simulink model "CHB_3phase_Phaseshift"  (R2015a)
settings: Solver=ode45  StartTime=0.0  StopTime=0.06  MaxStep=0.000001  MinStep=0.0000001  RelTol=1e-3
libraries: powerlib x33, powerlib_meascontrol x1, simulink x1
settings Model: Creator=hp  LastModifiedBy=hp

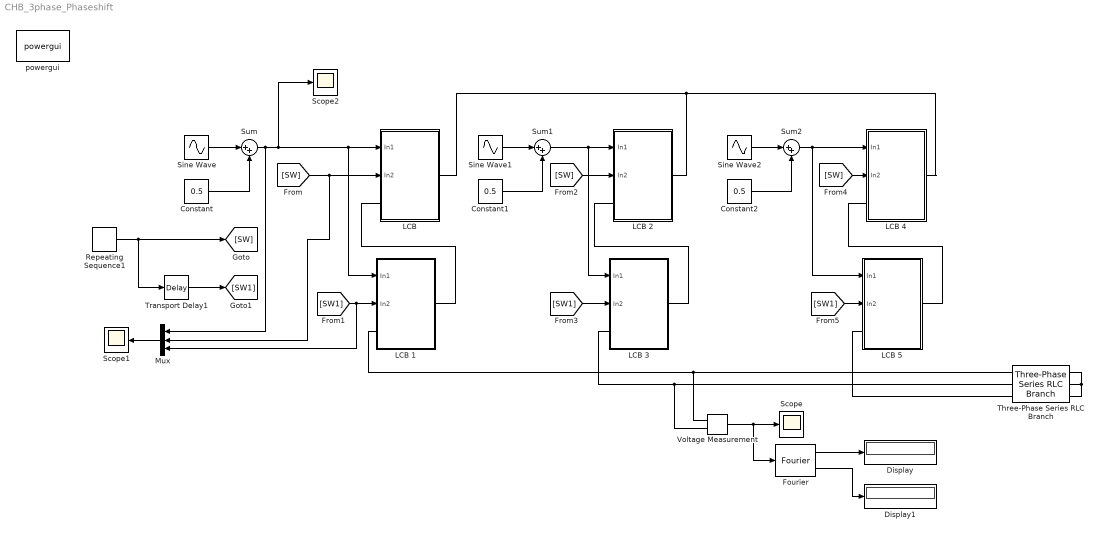
== system CHB_3phase_Phaseshift ==
  Constant : Constant  Value=0.5
  Constant1 : Constant  Value=0.5
  Constant2 : Constant  Value=0.5
  Display : Display
  Display1 : Display
  Fourier : powerlib_meascontrol/Measurements/Fourier  Freq=50  n=1  InInit=[0, 0]  Ts=0
  "LCB " : Subsystem
  LCB 1 : Subsystem
  LCB 2 : Subsystem
  LCB 3 : Subsystem
  LCB 4 : Subsystem
  LCB 5 : Subsystem
  Mux : Mux  Inputs=3
  Repeating Sequence1 : simulink/Sources/Repeating Sequence  rep_seq_t=[0 0.5 1]/1000  rep_seq_y=[0 1 0]
  Scope : Scope
      settings: YMin=-400  YMax=400
  Scope1 : Scope
      settings: YMin=2.77556e-17  YMax=1  SaveName=ScopeData2
  Scope2 : Scope
      settings: YMin=2.77556e-17  YMax=1  SaveName=ScopeData3
  Sine Wave : Sin  Amplitude=0.5  Frequency=2*pi*50  SampleTime=0
  Sine Wave1 : Sin  Amplitude=0.5  Frequency=2*pi*50  Phase=2*pi/3  SampleTime=0
  Sine Wave2 : Sin  Amplitude=0.5  Frequency=2*pi*50  Phase=4*pi/3  SampleTime=0
  Sum : Sum  Inputs=|++
  Sum1 : Sum  Inputs=|++
  Sum2 : Sum  Inputs=|++
  Three-Phase Series RLC Branch : powerlib/Elements/Three-Phase Series RLC Branch  LConnTagsString=A|B|C  RConnTagsString=A|B|C  BranchType=RLC  Resistance=1000  Inductance=0  Capacitance=0  Measurements=None
  Transport Delay1 : TransportDelay  DelayTime=1/4000
  Voltage Measurement : powerlib/Measurements/Voltage Measurement  PhasorSimulation=off  OutputType=Complex  PSBequivalent=0
  powergui : powerlib/powergui  Priority=1  SimulationMode=Continuous  SolverType=Tustin/Backward Euler (TBE)  SampleTime=50e-6  frequency=60  SPID=off  DisableSnubberDevices=off  DisableRonSwitches=off  DisableVfSwitches=off  SwTol=0  DisplayEquations=off  Interpol=off  methode=off  Ts=100  FunctionMessages=off  echomessages=off  HookPort=off  EnableUseOfTLC=off  x0status=blocks  frequencyindice=0  Pbase=100e6  ErrMax=1e-4  Iterations=50  UnitsV=kV  UnitsW=MW  buscounter=0  RestoreLinks=warning  ResistiveCurrentMeasurement=off  Frange=[0:2:500]  Ylog=off  Xlog=on  ShowGrid=off  save=off  variable=ZData  structure=0  ZoomFFT=off  StartTime=0.0  cycles=1  DisplayStyle=1  fundamental=60  FreqAxis=off  MaxFrequency=1000  frequencyindicesteady=1  RmsSteady=1  display=off
  wires:
  Sine Wave/1 -> Sum/1
  Sum/1 -> Mux/1, Scope2/1, LCB 1/1(In1), "LCB "/1(In1)
  Constant/1 -> Sum/2
  Mux/1 -> Scope1/1
  Sum1/1 -> LCB 3/1(In1), LCB 2/1(In1)
  [SW] -> LCB 2/2(In2)
  Repeating Sequence1/1 -> Transport Delay1/1, [SW]
  Transport Delay1/1 -> [SW1]
  [SW] -> Mux/2, "LCB "/2(In2)
  [SW1] -> LCB 1/2(In2), Mux/3
  [SW1] -> LCB 3/2(In2)
  Sine Wave1/1 -> Sum1/1
  Constant1/1 -> Sum1/2
  Sine Wave2/1 -> Sum2/1
  Constant2/1 -> Sum2/2
  Sum2/1 -> LCB 4/1(In1), LCB 5/1(In1)
  [SW] -> LCB 4/2(In2)
  [SW1] -> LCB 5/2(In2)
  Voltage Measurement/1 -> Fourier/1, Scope/1
  Fourier/1 -> Display/1
  Fourier/2 -> Display1/1
  connections:
  LCB 1/RConn1 -- "LCB "/LConn1
  LCB 3/RConn1 -- LCB 2/LConn1
  LCB 5/RConn1 -- LCB 4/LConn1
  Three-Phase Series RLC Branch/LConn1 -- Voltage Measurement/LConn1 -- LCB 1/LConn1
  Three-Phase Series RLC Branch/LConn2 -- Voltage Measurement/LConn2 -- LCB 3/LConn1
  Three-Phase Series RLC Branch/LConn3 -- LCB 5/LConn1
  Three-Phase Series RLC Branch/RConn1 -- Three-Phase Series RLC Branch/RConn2 -- Three-Phase Series RLC Branch/RConn3
  "LCB "/RConn1 -- LCB 4/RConn1 -- LCB 2/RConn1

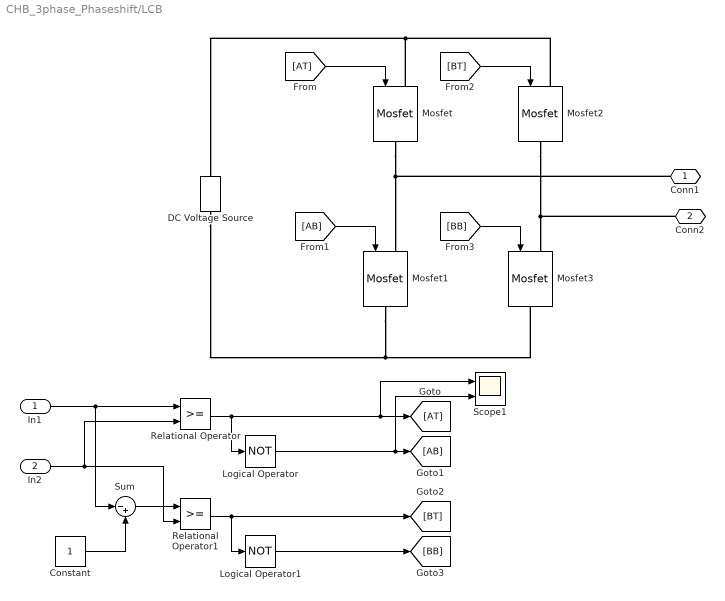
== system CHB_3phase_Phaseshift/LCB  ==
  In1 : Inport
  In2 : Inport  Port=2
  Constant : Constant
  DC Voltage Source : powerlib/Electrical Sources/DC Voltage Source  Amplitude=100  Measurements=None
  Logical Operator : Logic  Operator=NOT  Inputs=1  AllPortsSameDT=off  OutDataTypeStr=boolean
  Logical Operator1 : Logic  Operator=NOT  Inputs=1  AllPortsSameDT=off  OutDataTypeStr=boolean
  Mosfet{,1..3} (4 alike) : powerlib/Power Electronics/Mosfet  Ron=0.1  Lon=0  Rd=0.01  Vfd=0  IC=0  Rs=1e5  Cs=inf  Measurements=off
  Relational Operator : RelationalOperator  OutDataTypeStr=boolean
  Relational Operator1 : RelationalOperator  OutDataTypeStr=boolean
  Scope1 : Scope  NumInputPorts=2
      settings: YMin=-80~-5  YMax=80~5
  Sum : Sum  Inputs=|-+
  Conn1 : PMIOPort  Port=1  Side=Right
  Conn2 : PMIOPort  Port=2  Side=Left
  wires:
  Sum/1 -> Relational Operator1/1
  Relational Operator/1 -> Scope1/1, [AT], Logical Operator/1
  Logical Operator/1 -> Scope1/2, [AB]
  Relational Operator1/1 -> [BT], Logical Operator1/1
  Logical Operator1/1 -> [BB]
  [BB] -> Mosfet3/1
  [AB] -> Mosfet1/1
  [AT] -> Mosfet/1
  [BT] -> Mosfet2/1
  In2/1 -> Relational Operator1/2, Relational Operator/2
  In1/1 -> Sum/1, Relational Operator/1
  Constant/1 -> Sum/2
  connections:
  Mosfet2/RConn1 -- Conn2/RConn1 -- Mosfet3/LConn1
  DC Voltage Source/LConn1 -- Mosfet1/RConn1 -- Mosfet3/RConn1
  Mosfet2/LConn1 -- Mosfet/LConn1 -- DC Voltage Source/RConn1
  Mosfet/RConn1 -- Conn1/RConn1 -- Mosfet1/LConn1

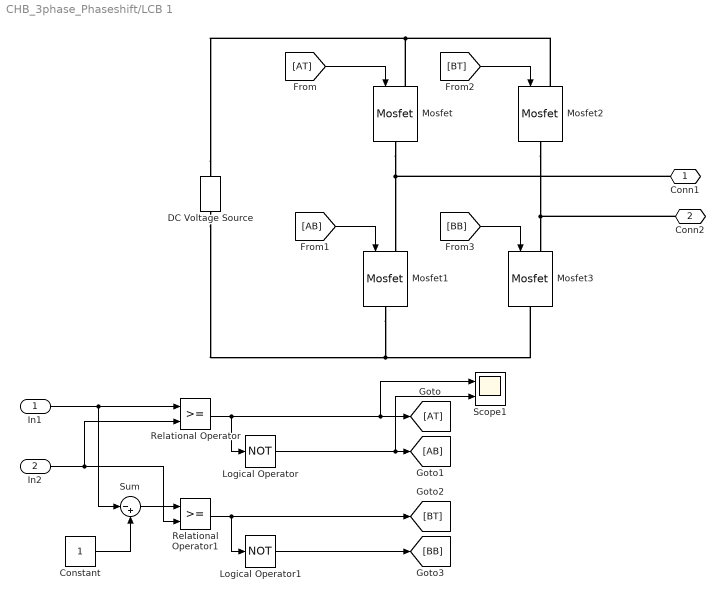
== system CHB_3phase_Phaseshift/LCB 1 ==
  In1 : Inport
  In2 : Inport  Port=2
  Constant : Constant
  DC Voltage Source : powerlib/Electrical Sources/DC Voltage Source  Amplitude=100  Measurements=None
  Logical Operator : Logic  Operator=NOT  Inputs=1  AllPortsSameDT=off  OutDataTypeStr=boolean
  Logical Operator1 : Logic  Operator=NOT  Inputs=1  AllPortsSameDT=off  OutDataTypeStr=boolean
  Mosfet{,1..3} (4 alike) : powerlib/Power Electronics/Mosfet  Ron=0.1  Lon=0  Rd=0.01  Vfd=0  IC=0  Rs=1e5  Cs=inf  Measurements=off
  Relational Operator : RelationalOperator  OutDataTypeStr=boolean
  Relational Operator1 : RelationalOperator  OutDataTypeStr=boolean
  Scope1 : Scope  NumInputPorts=2
      settings: YMin=-80~-5  YMax=80~5
  Sum : Sum  Inputs=|-+
  Conn1 : PMIOPort  Port=1  Side=Right
  Conn2 : PMIOPort  Port=2  Side=Left
  wires:
  Sum/1 -> Relational Operator1/1
  Relational Operator/1 -> Scope1/1, [AT], Logical Operator/1
  Logical Operator/1 -> Scope1/2, [AB]
  Relational Operator1/1 -> [BT], Logical Operator1/1
  Logical Operator1/1 -> [BB]
  [BB] -> Mosfet3/1
  [AB] -> Mosfet1/1
  [AT] -> Mosfet/1
  [BT] -> Mosfet2/1
  In2/1 -> Relational Operator1/2, Relational Operator/2
  In1/1 -> Sum/1, Relational Operator/1
  Constant/1 -> Sum/2
  connections:
  Mosfet2/RConn1 -- Conn2/RConn1 -- Mosfet3/LConn1
  Mosfet3/RConn1 -- DC Voltage Source/LConn1 -- Mosfet1/RConn1
  DC Voltage Source/RConn1 -- Mosfet2/LConn1 -- Mosfet/LConn1
  Mosfet/RConn1 -- Mosfet1/LConn1 -- Conn1/RConn1

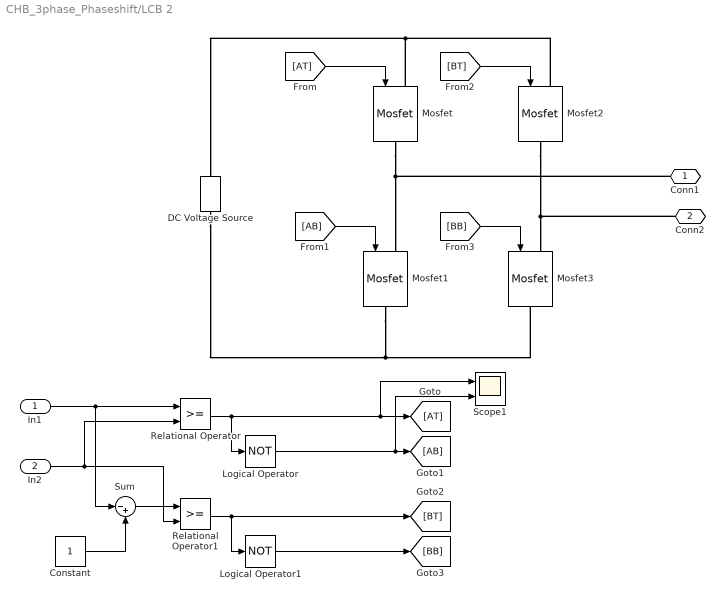
== system CHB_3phase_Phaseshift/LCB 2 ==
  In1 : Inport
  In2 : Inport  Port=2
  Constant : Constant
  DC Voltage Source : powerlib/Electrical Sources/DC Voltage Source  Amplitude=100  Measurements=None
  Logical Operator : Logic  Operator=NOT  Inputs=1  AllPortsSameDT=off  OutDataTypeStr=boolean
  Logical Operator1 : Logic  Operator=NOT  Inputs=1  AllPortsSameDT=off  OutDataTypeStr=boolean
  Mosfet{,1..3} (4 alike) : powerlib/Power Electronics/Mosfet  Ron=0.1  Lon=0  Rd=0.01  Vfd=0  IC=0  Rs=1e5  Cs=inf  Measurements=off
  Relational Operator : RelationalOperator  OutDataTypeStr=boolean
  Relational Operator1 : RelationalOperator  OutDataTypeStr=boolean
  Scope1 : Scope  NumInputPorts=2
      settings: YMin=-80~-5  YMax=80~5
  Sum : Sum  Inputs=|-+
  Conn1 : PMIOPort  Port=1  Side=Right
  Conn2 : PMIOPort  Port=2  Side=Left
  wires:
  Sum/1 -> Relational Operator1/1
  Relational Operator/1 -> Scope1/1, [AT], Logical Operator/1
  Logical Operator/1 -> Scope1/2, [AB]
  Relational Operator1/1 -> [BT], Logical Operator1/1
  Logical Operator1/1 -> [BB]
  [BB] -> Mosfet3/1
  [AB] -> Mosfet1/1
  [AT] -> Mosfet/1
  [BT] -> Mosfet2/1
  In2/1 -> Relational Operator1/2, Relational Operator/2
  In1/1 -> Sum/1, Relational Operator/1
  Constant/1 -> Sum/2
  connections:
  Mosfet2/RConn1 -- Conn2/RConn1 -- Mosfet3/LConn1
  DC Voltage Source/LConn1 -- Mosfet1/RConn1 -- Mosfet3/RConn1
  Mosfet2/LConn1 -- Mosfet/LConn1 -- DC Voltage Source/RConn1
  Mosfet/RConn1 -- Conn1/RConn1 -- Mosfet1/LConn1

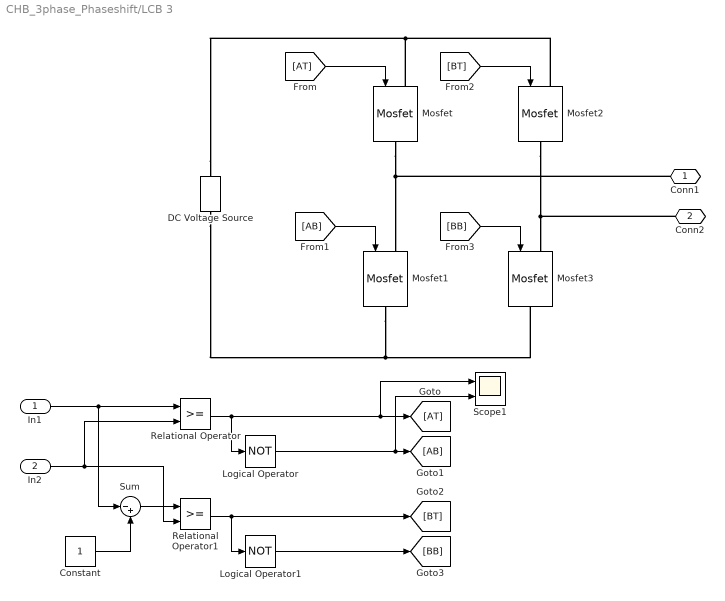
== system CHB_3phase_Phaseshift/LCB 3 ==
  In1 : Inport
  In2 : Inport  Port=2
  Constant : Constant
  DC Voltage Source : powerlib/Electrical Sources/DC Voltage Source  Amplitude=100  Measurements=None
  Logical Operator : Logic  Operator=NOT  Inputs=1  AllPortsSameDT=off  OutDataTypeStr=boolean
  Logical Operator1 : Logic  Operator=NOT  Inputs=1  AllPortsSameDT=off  OutDataTypeStr=boolean
  Mosfet{,1..3} (4 alike) : powerlib/Power Electronics/Mosfet  Ron=0.1  Lon=0  Rd=0.01  Vfd=0  IC=0  Rs=1e5  Cs=inf  Measurements=off
  Relational Operator : RelationalOperator  OutDataTypeStr=boolean
  Relational Operator1 : RelationalOperator  OutDataTypeStr=boolean
  Scope1 : Scope  NumInputPorts=2
      settings: YMin=-80~-5  YMax=80~5
  Sum : Sum  Inputs=|-+
  Conn1 : PMIOPort  Port=1  Side=Right
  Conn2 : PMIOPort  Port=2  Side=Left
  wires:
  Sum/1 -> Relational Operator1/1
  Relational Operator/1 -> Scope1/1, [AT], Logical Operator/1
  Logical Operator/1 -> Scope1/2, [AB]
  Relational Operator1/1 -> [BT], Logical Operator1/1
  Logical Operator1/1 -> [BB]
  [BB] -> Mosfet3/1
  [AB] -> Mosfet1/1
  [AT] -> Mosfet/1
  [BT] -> Mosfet2/1
  In2/1 -> Relational Operator1/2, Relational Operator/2
  In1/1 -> Sum/1, Relational Operator/1
  Constant/1 -> Sum/2
  connections:
  Mosfet2/RConn1 -- Conn2/RConn1 -- Mosfet3/LConn1
  Mosfet3/RConn1 -- DC Voltage Source/LConn1 -- Mosfet1/RConn1
  DC Voltage Source/RConn1 -- Mosfet2/LConn1 -- Mosfet/LConn1
  Mosfet/RConn1 -- Mosfet1/LConn1 -- Conn1/RConn1

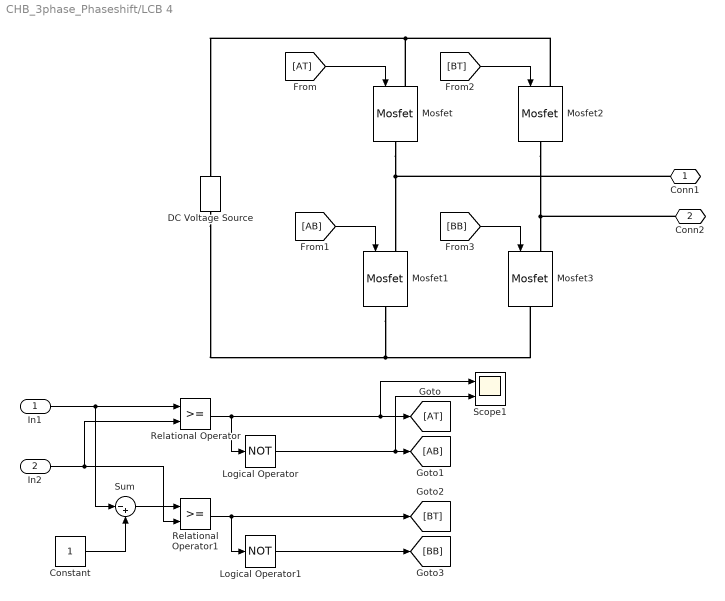
== system CHB_3phase_Phaseshift/LCB 4 ==
  In1 : Inport
  In2 : Inport  Port=2
  Constant : Constant
  DC Voltage Source : powerlib/Electrical Sources/DC Voltage Source  Amplitude=100  Measurements=None
  Logical Operator : Logic  Operator=NOT  Inputs=1  AllPortsSameDT=off  OutDataTypeStr=boolean
  Logical Operator1 : Logic  Operator=NOT  Inputs=1  AllPortsSameDT=off  OutDataTypeStr=boolean
  Mosfet{,1..3} (4 alike) : powerlib/Power Electronics/Mosfet  Ron=0.1  Lon=0  Rd=0.01  Vfd=0  IC=0  Rs=1e5  Cs=inf  Measurements=off
  Relational Operator : RelationalOperator  OutDataTypeStr=boolean
  Relational Operator1 : RelationalOperator  OutDataTypeStr=boolean
  Scope1 : Scope  NumInputPorts=2
      settings: YMin=-80~-5  YMax=80~5
  Sum : Sum  Inputs=|-+
  Conn1 : PMIOPort  Port=1  Side=Right
  Conn2 : PMIOPort  Port=2  Side=Left
  wires:
  Sum/1 -> Relational Operator1/1
  Relational Operator/1 -> Scope1/1, [AT], Logical Operator/1
  Logical Operator/1 -> Scope1/2, [AB]
  Relational Operator1/1 -> [BT], Logical Operator1/1
  Logical Operator1/1 -> [BB]
  [BB] -> Mosfet3/1
  [AB] -> Mosfet1/1
  [AT] -> Mosfet/1
  [BT] -> Mosfet2/1
  In2/1 -> Relational Operator1/2, Relational Operator/2
  In1/1 -> Sum/1, Relational Operator/1
  Constant/1 -> Sum/2
  connections:
  Mosfet2/RConn1 -- Conn2/RConn1 -- Mosfet3/LConn1
  DC Voltage Source/LConn1 -- Mosfet1/RConn1 -- Mosfet3/RConn1
  Mosfet2/LConn1 -- Mosfet/LConn1 -- DC Voltage Source/RConn1
  Mosfet/RConn1 -- Conn1/RConn1 -- Mosfet1/LConn1

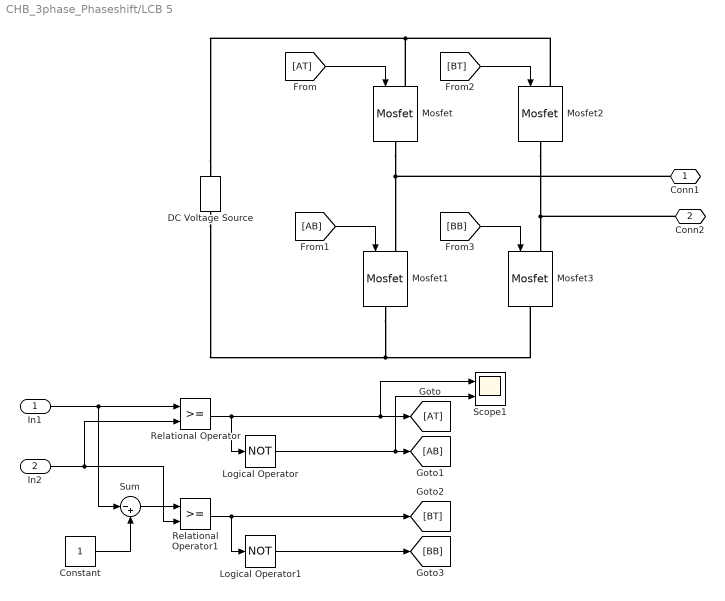
== system CHB_3phase_Phaseshift/LCB 5 ==
  In1 : Inport
  In2 : Inport  Port=2
  Constant : Constant
  DC Voltage Source : powerlib/Electrical Sources/DC Voltage Source  Amplitude=100  Measurements=None
  Logical Operator : Logic  Operator=NOT  Inputs=1  AllPortsSameDT=off  OutDataTypeStr=boolean
  Logical Operator1 : Logic  Operator=NOT  Inputs=1  AllPortsSameDT=off  OutDataTypeStr=boolean
  Mosfet{,1..3} (4 alike) : powerlib/Power Electronics/Mosfet  Ron=0.1  Lon=0  Rd=0.01  Vfd=0  IC=0  Rs=1e5  Cs=inf  Measurements=off
  Relational Operator : RelationalOperator  OutDataTypeStr=boolean
  Relational Operator1 : RelationalOperator  OutDataTypeStr=boolean
  Scope1 : Scope  NumInputPorts=2
      settings: YMin=-80~-5  YMax=80~5
  Sum : Sum  Inputs=|-+
  Conn1 : PMIOPort  Port=1  Side=Right
  Conn2 : PMIOPort  Port=2  Side=Left
  wires:
  Sum/1 -> Relational Operator1/1
  Relational Operator/1 -> Scope1/1, [AT], Logical Operator/1
  Logical Operator/1 -> Scope1/2, [AB]
  Relational Operator1/1 -> [BT], Logical Operator1/1
  Logical Operator1/1 -> [BB]
  [BB] -> Mosfet3/1
  [AB] -> Mosfet1/1
  [AT] -> Mosfet/1
  [BT] -> Mosfet2/1
  In2/1 -> Relational Operator1/2, Relational Operator/2
  In1/1 -> Sum/1, Relational Operator/1
  Constant/1 -> Sum/2
  connections:
  Mosfet2/RConn1 -- Conn2/RConn1 -- Mosfet3/LConn1
  Mosfet3/RConn1 -- DC Voltage Source/LConn1 -- Mosfet1/RConn1
  DC Voltage Source/RConn1 -- Mosfet2/LConn1 -- Mosfet/LConn1
  Mosfet/RConn1 -- Mosfet1/LConn1 -- Conn1/RConn1
